simulink model "SecondOrderSystemAdjustment"  (R2013b)
settings: Solver=ode45  StartTime=0.0  StopTime=50  RelTol=1e-3
settings Model: Creator=MMSA  LastModifiedBy=MMSA
settings SolverCC: ZeroCrossAlgorithm=Adaptive  PositivePriorityOrder=on
settings HardwareCC: ProdBitPerPointer=64  ProdHWDeviceType=Generic->64-bit Embedded Processor (LLP64)

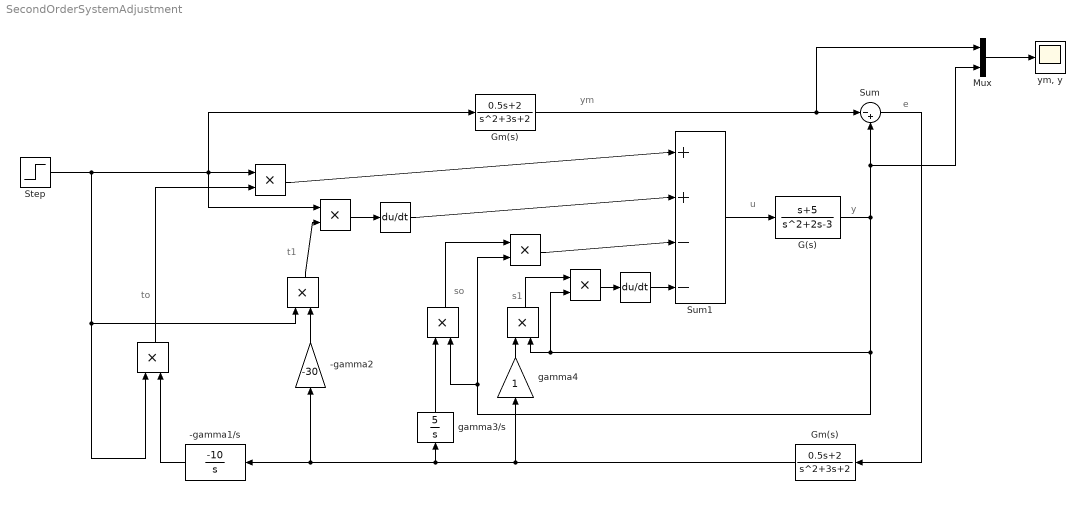
== system SecondOrderSystemAdjustment ==
  note: e
  note: y
  note: u
  note: s1
  note: so
  note: ym
  note: t1
  note: to
   {,,,,} (5 alike) : Product
  "   " : Product
  "    " : Product
  " " : Derivative
  " " : Derivative
  "         " : Product
  -gamma1/s : TransferFcn  Numerator=[-10]  Denominator=[1 0]
  -gamma2 : Gain  Gain=-30
  G(s) : TransferFcn  Numerator=[1 5]  Denominator=[1 2 -3]
  Gm(s) : TransferFcn  Numerator=[0.5 2]  Denominator=[1 3 2]
  "Gm(s) " : TransferFcn  Numerator=[0.5 2]  Denominator=[1 3 2]
  Mux : Mux  Inputs=2
  Step : Step  Time=0  SampleTime=0
  Sum : Sum  Inputs=|-+
  Sum1 : Sum  Inputs=|++--
  gamma3/s : TransferFcn  Numerator=[5]  Denominator=[1 0]
  gamma4 : Gain
  "ym, y" : Scope
      settings: TimeRange=6.000000496442226e-10  YMin=0.9500000000000001  YMax=1.3
  wires:
  Mux/1 -> "ym, y"/1
  Gm(s)/1 -> Mux/1, Sum/1
  G(s)/1 -> " "/2, " "/2, " "/2, "         "/2, Sum/2, Mux/2
  Sum/1 -> "Gm(s) "/1
  Step/1 -> " "/1, "    "/1, " "/1, Gm(s)/1, "   "/1
  Sum1/1 -> G(s)/1
  "   "/1 -> Sum1/1
  "Gm(s) "/1 -> gamma4/1, -gamma1/s/1, -gamma2/1, gamma3/s/1
  -gamma1/s/1 -> " "/2
  " "/1 -> "   "/2
  -gamma2/1 -> "    "/2
  " "/1 -> " "/1
  "    "/1 -> " "/2
  " "/1 -> Sum1/2
  gamma3/s/1 -> "         "/1
  "         "/1 -> " "/1
  " "/1 -> Sum1/3
  gamma4/1 -> " "/1
  " "/1 -> " "/1
  " "/1 -> " "/1
  " "/1 -> Sum1/4
